simulink model "velocityControl"  (R2020b)
settings: Solver=VariableStepAuto  StartTime=0.0  StopTime=20.0  RelTol=1e-3
values from neighbouring files (symbols this model uses):
  condtheta = x0(3)    [MPCdefinition.m]
  condx = x0(1)    [MPCdefinition.m]
  condy = x0(2)    [MPCdefinition.m]
  k_obsx = 2    [MPCdefinition.m]
  k_obsy = 2    [MPCdefinition.m]
  omega_max_perc = 0.1    [MPCdefinition.m]
  omega_min_perc = -0.1    [MPCdefinition.m]
  v_max_perc = 0.5    [MPCdefinition.m]
  v_min_perc = -0.5    [MPCdefinition.m]
libraries: mpclib x1
settings Model: Creator=adelina  LastModifiedBy=adelina

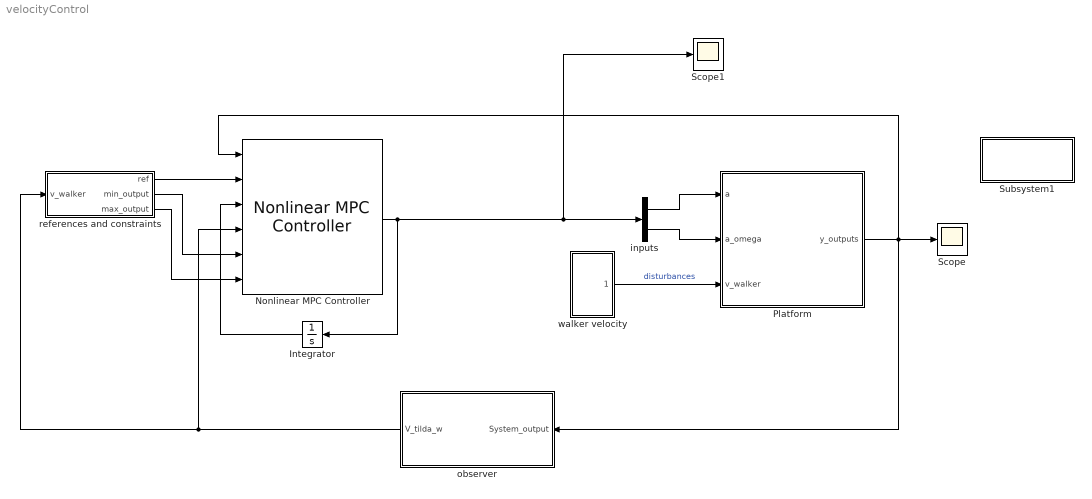
== system velocityControl ==
  Integrator : Integrator
  Nonlinear MPC Controller : mpclib/Nonlinear MPC Controller  SCDEnableBlockLinearizationSpecification=on  nlmpcobj=nlobj  UseObjectTs=on  UseMEX=off  md_enabled=on  mvtarget_enabled=off  param_enabled=off  cost_enabled=off  mvseq_enabled=off  stateseq_enabled=off  ovseq_enabled=off  slack_enabled=off  status_enabled=off  ov_min=on  ov_max=on  mv_min=off  mv_max=off  mvrate_min=off  mvrate_max=off  state_min=off  state_max=off  ov_weight=off  mv_weight=off  mvrate_weight=off  ecr_weight=off  nlp_initialize=off
  Platform : Subsystem
  Scope : Scope
  Scope1 : Scope
  Subsystem1 : Subsystem
      settings: OpenFcn=plots
      mask Display: disp('plots')
  inputs : Demux  Outputs=2
  observer : Subsystem
  references and constraints : Subsystem
  walker velocity : Subsystem
  wires:
  Nonlinear MPC Controller/1 -> Scope1/1, inputs/1, Integrator/1
  inputs/2 -> Platform/2(a_omega)
  inputs/1 -> Platform/1(a)
  Integrator/1 -> Nonlinear MPC Controller/3
  references and constraints/1(ref) -> Nonlinear MPC Controller/2
  Platform/1(y_outputs) -> observer/1(System_output), Scope/1, Nonlinear MPC Controller/1
  walker velocity/1(v_walker) -> Platform/3(v_walker)  "disturbances"
  observer/1(V_tilda_w) -> Nonlinear MPC Controller/4, references and constraints/1(v_walker)
  references and constraints/2(min_output) -> Nonlinear MPC Controller/5
  references and constraints/3(max_output) -> Nonlinear MPC Controller/6

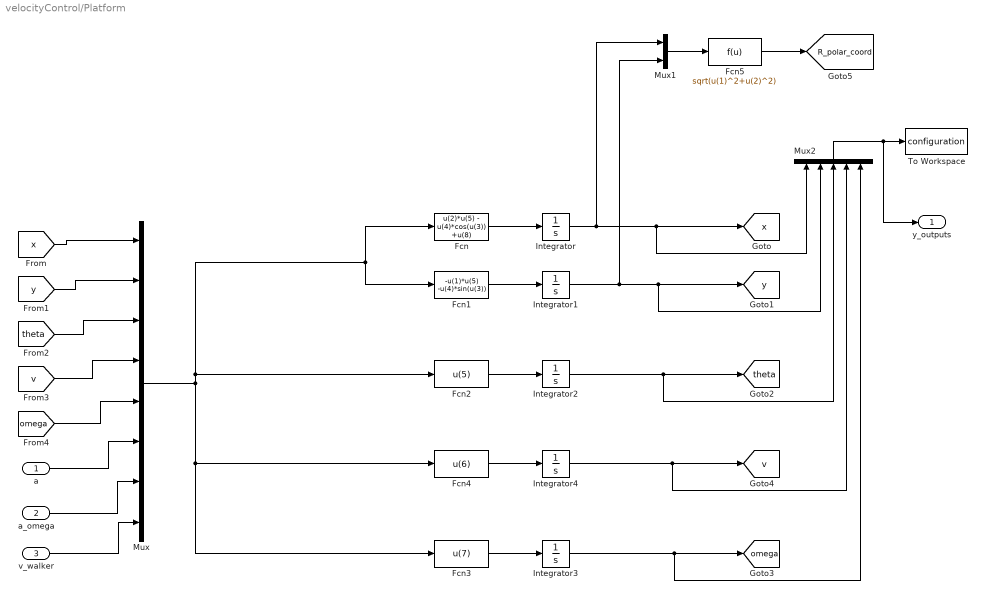
== system velocityControl/Platform ==
  a : Inport
  a_omega : Inport  Port=2
  v_walker : Inport  Port=3
  Fcn : Fcn  Expr=u(2)*u(5) - u(4)*cos(u(3)) +u(8)
  Fcn1 : Fcn  Expr=-u(1)*u(5) -u(4)*sin(u(3))
  Fcn2 : Fcn  Expr=u(5)
  Fcn3 : Fcn  Expr=u(7)
  Fcn4 : Fcn  Expr=u(6)
  Fcn5 : Fcn  Expr=sqrt(u(1)^2+u(2)^2)
  Integrator : Integrator  InitialCondition=condx
  Integrator1 : Integrator  InitialCondition=condy
  Integrator2 : Integrator  InitialCondition=condtheta
  Integrator3 : Integrator
  Integrator4 : Integrator
  Mux : Mux  Inputs=8
  Mux1 : Mux  Inputs=2
  Mux2 : Mux  Inputs=5
  To Workspace : ToWorkspace  VariableName=configuration  SaveFormat=Structure With Time  SampleTime=-1
  y_outputs : Outport
  tag scope: R_polar_coord=global, omega=global, theta=global, v=global, x=global, y=global
  wires:
  Fcn2/1 -> Integrator2/1
  Integrator2/1 -> [theta], Mux2/3
  Fcn1/1 -> Integrator1/1
  [y] -> Mux/2
  [x] -> Mux/1
  a/1 -> Mux/6
  Integrator1/1 -> Mux1/2, [y], Mux2/2
  [theta] -> Mux/3
  Integrator/1 -> Mux1/1, Mux2/1, [x]
  Fcn/1 -> Integrator/1
  a_omega/1 -> Mux/7
  Mux2/1 -> y_outputs/1, To Workspace/1
  [v] -> Mux/4
  [omega] -> Mux/5
  Mux/1 -> Fcn1/1, Fcn/1, Fcn2/1, Fcn3/1, Fcn4/1
  Integrator3/1 -> [omega], Mux2/5
  Fcn3/1 -> Integrator3/1
  Integrator4/1 -> Mux2/4, [v]
  Fcn4/1 -> Integrator4/1
  v_walker/1 -> Mux/8
  Mux1/1 -> Fcn5/1
  Fcn5/1 -> [R_polar_coord]

== system velocityControl/Subsystem1 ==

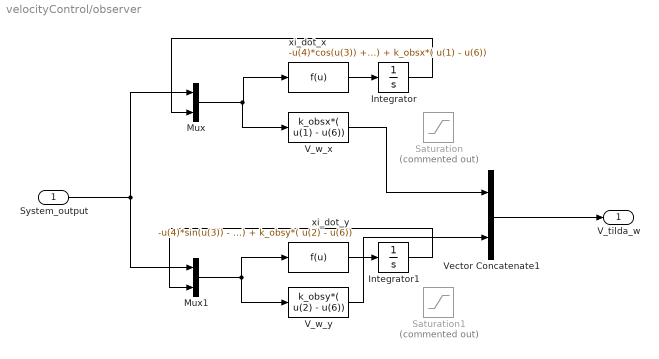
== system velocityControl/observer ==
  System_output : Inport
  Integrator : Integrator  InitialCondition=condx
  Integrator1 : Integrator  InitialCondition=condy
  Mux : Mux  Inputs=2
  Mux1 : Mux  Inputs=2
  Saturation : Saturate  Commented=on
  Saturation1 : Saturate  Commented=on
  V_w_x : Fcn  Expr=k_obsx*( u(1) - u(6))
  V_w_y : Fcn  Expr=k_obsy*( u(2) - u(6))
  Vector Concatenate1 : Concatenate  Mode=Multidimensional array  ConcatenateDimension=2
  xi_dot_x : Fcn  Expr=-u(4)*cos(u(3)) + u(2)*u(5) + k_obsx*( u(1) - u(6))
  xi_dot_y : Fcn  Expr=-u(4)*sin(u(3)) - u(1)*u(5) + k_obsy*( u(2) - u(6))
  V_tilda_w : Outport
  wires:
  Mux/1 -> V_w_x/1, xi_dot_x/1
  Mux1/1 -> V_w_y/1, xi_dot_y/1
  System_output/1 -> Mux/1, Mux1/1
  Vector Concatenate1/1 -> V_tilda_w/1
  xi_dot_x/1 -> Integrator/1
  Integrator/1 -> Mux/2
  xi_dot_y/1 -> Integrator1/1
  Integrator1/1 -> Mux1/2
  V_w_y/1 -> Vector Concatenate1/2
  V_w_x/1 -> Vector Concatenate1/1

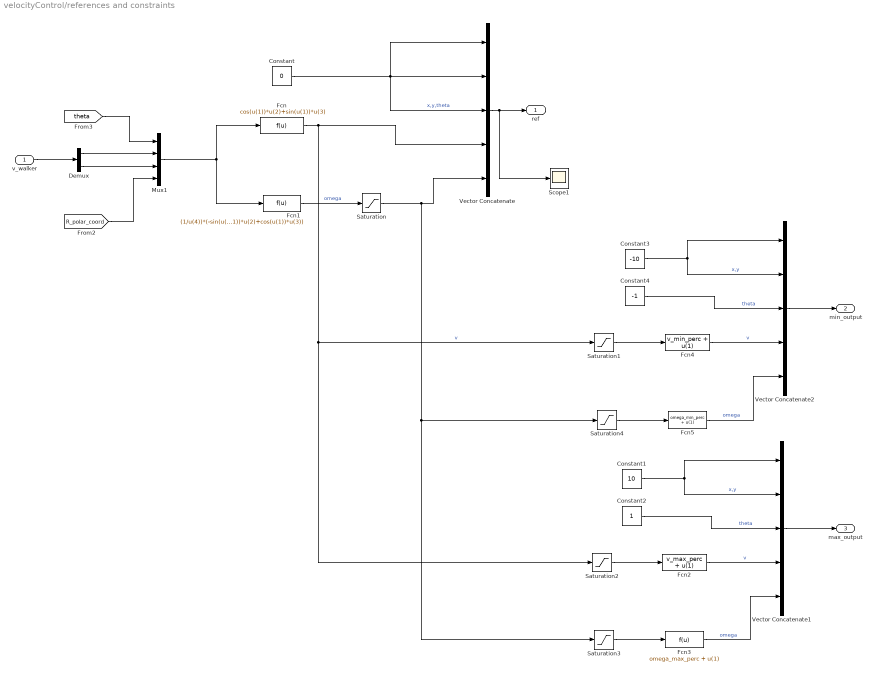
== system velocityControl/references and constraints ==
  v_walker : Inport
  Constant : Constant  Value=0
  Constant1 : Constant  Value=10
  Constant2 : Constant
  Constant3 : Constant  Value=-10
  Constant4 : Constant  Value=-1
  Demux : Demux  Outputs=2
  Fcn : Fcn  Expr=cos(u(1))*u(2)+sin(u(1))*u(3)
  Fcn1 : Fcn  Expr=(1/u(4))*(-sin(u(1))*u(2)+cos(u(1))*u(3))
  Fcn2 : Fcn  Expr=v_max_perc + u(1)
  Fcn3 : Fcn  Expr=omega_max_perc + u(1)
  Fcn4 : Fcn  Expr=v_min_perc + u(1)
  Fcn5 : Fcn  Expr=omega_min_perc + u(1)
  Mux1 : Mux
  Saturation : Saturate  UpperLimit=0.1  LowerLimit=-0.1
  Saturation1 : Saturate  UpperLimit=0  LowerLimit=-inf
  Saturation2 : Saturate  UpperLimit=inf  LowerLimit=0
  Saturation3 : Saturate  UpperLimit=inf  LowerLimit=0
  Saturation4 : Saturate  UpperLimit=0  LowerLimit=-inf
  Scope1 : Scope
  Vector Concatenate : Concatenate  NumInputs=5  Mode=Multidimensional array  ConcatenateDimension=2
  Vector Concatenate1 : Concatenate  NumInputs=5  Mode=Multidimensional array  ConcatenateDimension=2
  Vector Concatenate2 : Concatenate  NumInputs=5  Mode=Multidimensional array  ConcatenateDimension=2
  ref : Outport
  min_output : Outport  Port=2
  max_output : Outport  Port=3
  wires:
  Constant/1 -> Vector Concatenate/1, Vector Concatenate/3, Vector Concatenate/2  "x,y,theta"
  Vector Concatenate/1 -> Scope1/1, ref/1
  [R_polar_coord] -> Mux1/4
  [theta] -> Mux1/1
  Demux/1 -> Mux1/2
  Demux/2 -> Mux1/3
  Fcn1/1 -> Saturation/1  "omega"
  Fcn2/1 -> Vector Concatenate1/4  "v"
  Constant1/1 -> Vector Concatenate1/2, Vector Concatenate1/1  "x,y"
  Mux1/1 -> Fcn/1, Fcn1/1
  Fcn3/1 -> Vector Concatenate1/5  "omega"
  Constant2/1 -> Vector Concatenate1/3  "theta"
  Saturation2/1 -> Fcn2/1
  Saturation3/1 -> Fcn3/1
  Fcn5/1 -> Vector Concatenate2/5  "omega"
  Constant4/1 -> Vector Concatenate2/3  "theta"
  Saturation/1 -> Saturation3/1, Saturation4/1, Vector Concatenate/5
  Fcn/1 -> Saturation2/1, Saturation1/1, Vector Concatenate/4  "v"
  Fcn4/1 -> Vector Concatenate2/4  "v"
  Saturation4/1 -> Fcn5/1
  Saturation1/1 -> Fcn4/1
  Constant3/1 -> Vector Concatenate2/2, Vector Concatenate2/1  "x,y"
  Vector Concatenate2/1 -> min_output/1
  Vector Concatenate1/1 -> max_output/1
  v_walker/1 -> Demux/1

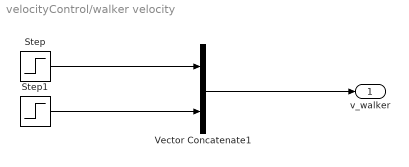
== system velocityControl/walker velocity ==
  Step : Step  Time=20  After=0.2  SampleTime=0
  Step1 : Step  Time=10  After=0.1  SampleTime=0
  Vector Concatenate1 : Concatenate  Mode=Multidimensional array  ConcatenateDimension=2
  v_walker : Outport
  wires:
  Step1/1 -> Vector Concatenate1/2
  Vector Concatenate1/1 -> v_walker/1
  Step/1 -> Vector Concatenate1/1
